simulink model "test"  (R2024a)
settings: Solver=VariableStepAuto  StartTime=0.0  StopTime=10.0  RelTol=1e-3
values from neighbouring files (symbols this model uses):
  U = [50; 60]    [main.m]
undefined symbols (not defined in the file or in its folder): A_bar, B_bar
libraries: cstblocks x1
settings Model: Creator=scott  LastModifiedBy=scott

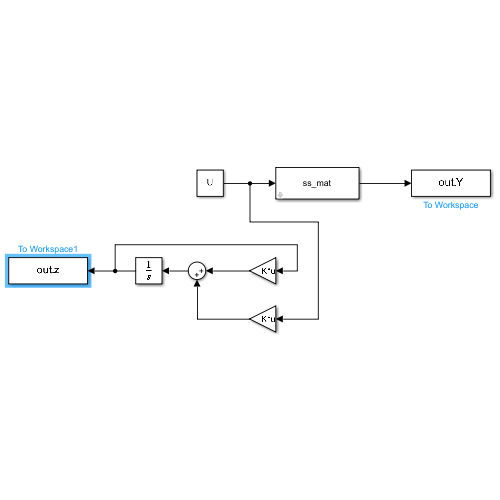
[thumbnail: Simulink's stored preview of the top-level diagram]
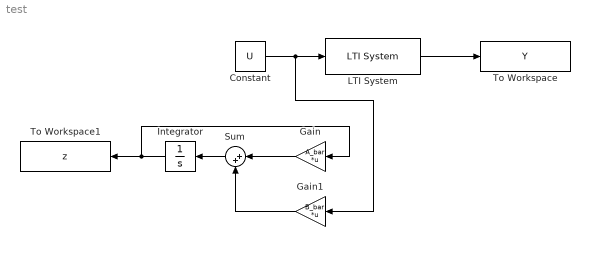
== system test ==
  Constant : Constant  Value=U
  Gain : Gain  Gain=A_bar  Multiplication=Matrix(K*u)
  Gain1 : Gain  Gain=B_bar  Multiplication=Matrix(K*u)
  Integrator : Integrator
  LTI System : cstblocks/LTI System  sys=ss_mat  IC=[]  PadeOrder=0
  Sum : Sum  Inputs=|++
  To Workspace : ToWorkspace  VariableName=Y  SaveFormat=Structure With Time  SampleTime=-1
  To Workspace1 : ToWorkspace  VariableName=z  SaveFormat=Structure  SampleTime=-1
  wires:
  Constant/1 -> Gain1/1, LTI System/1
  LTI System/1 -> To Workspace/1
  Gain/1 -> Sum/1
  Sum/1 -> Integrator/1
  Integrator/1 -> To Workspace1/1, Gain/1
  Gain1/1 -> Sum/2
